simulink model "FeedBack_Linearization"  (R2021b)
settings: Solver=VariableStepAuto  StartTime=0.0  StopTime=10.0  RelTol=1e-3
undefined symbols (not defined in the file): Kd, Kp, q_dq_init
(part 1 of 9)
settings Model: Creator=Yafei Ou  LastModifiedBy=Kirill

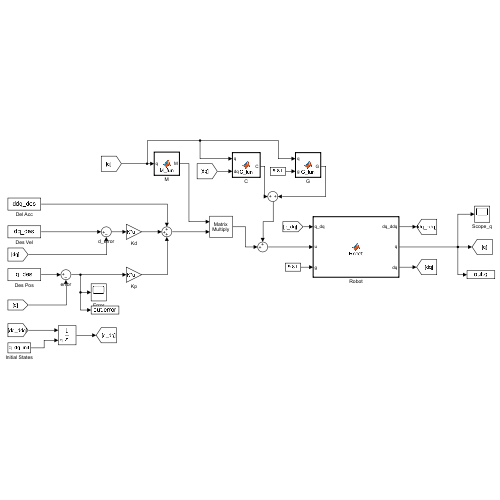
[thumbnail: Simulink's stored preview of the top-level diagram]
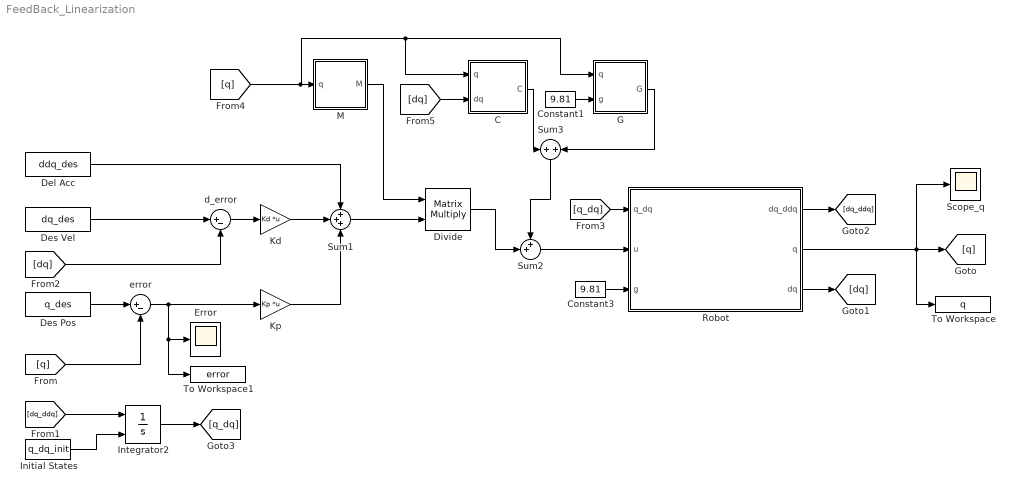
== system FeedBack_Linearization ==
  C : MATLAB Function  TreatAsAtomicUnit=on
  Constant1 : Constant  Value=9.81
  Constant3 : Constant  Value=9.81
  Del Acc : FromWorkspace  VariableName=ddq_des
  Des Pos : FromWorkspace  VariableName=q_des
  Des Vel : FromWorkspace  VariableName=dq_des
  Divide : Product  Inputs=**  Multiplication=Matrix(*)
  Error : Scope
  G : MATLAB Function  TreatAsAtomicUnit=on
  Initial States : Constant  Value=q_dq_init
  Integrator2 : Integrator  InitialConditionSource=external
  Kd : Gain  Gain=Kd  Multiplication=Matrix(K*u)
  Kp : Gain  Gain=Kp  Multiplication=Matrix(K*u)
  M : MATLAB Function  TreatAsAtomicUnit=on
  Robot : MATLAB Function  TreatAsAtomicUnit=on
  Scope_q : Scope
  Sum1 : Sum  Inputs=+++
  Sum2 : Sum  Inputs=++|
  Sum3 : Sum  Inputs=+|+
  To Workspace : ToWorkspace  VariableName=q  SaveFormat=Timeseries  SampleTime=-1
  To Workspace1 : ToWorkspace  VariableName=error  SaveFormat=Timeseries  SampleTime=-1
  d_error : Sum  Inputs=|+-
  error : Sum  Inputs=|+-
  wires:
  M/1(M) -> Divide/1
  C/1(C) -> Sum3/1
  Kp/1 -> Sum1/3
  Divide/1 -> Sum2/2
  Kd/1 -> Sum1/2
  Des Vel/1 -> d_error/1
  Sum1/1 -> Divide/2
  Constant1/1 -> G/2(g)
  d_error/1 -> Kd/1
  Des Pos/1 -> error/1
  G/1(G) -> Sum3/2
  Sum3/1 -> Sum2/1
  Del Acc/1 -> Sum1/1
  Sum2/1 -> Robot/2(u)
  error/1 -> To Workspace1/1, Error/1, Kp/1
  Constant3/1 -> Robot/3(g)
  Robot/2(q) -> Scope_q/1, To Workspace/1, [q]
  Robot/3(dq) -> [dq]
  Robot/1(dq_ddq) -> [dq_ddq]
  [q] -> error/2
  Initial States/1 -> Integrator2/2
  [dq_ddq] -> Integrator2/1
  Integrator2/1 -> [q_dq]
  [dq] -> d_error/2
  [q_dq] -> Robot/1(q_dq)
  [q] -> G/1(q), C/1(q), M/1(q)
  [dq] -> C/2(dq)
